simulink model "qrd_matrix_inversion"  (Simulink 8.7)
settings: Solver=VariableStepDiscrete  StartTime=0.0  StopTime=10  RelTol=1e-3
undefined symbols (not defined in the file or in its folder): dspba, Input_Fraction_Length, Input_Word_Length, value
libraries: DSPBAPrim x28, DSPBABase x6, qrd_matrix_library x1
Description:
  | DSP Builder Advanced Template for Template Design implementing Primitive Subsystems
settings Model: Creator=mjervis  LastModifiedBy=5g
settings DataIOCC: SignalLoggingSaveFormat=ModelDataLogs
settings OptimizationCC: ExpressionDepthLimit=2147483647
settings DebuggingCC: SolverPrmCheckMsg=warning  InheritedTsInSrcMsg=none  IntegerOverflowMsg=none  FcnCallInpInsideContextMsg=UseLocalSettings  AllowSymbolicDim=off  StateNameClashWarn=warning  IntegerSaturationMsg=none
settings GRTTargetCC: CombineOutputUpdateFcns=off  GRTInterface=on

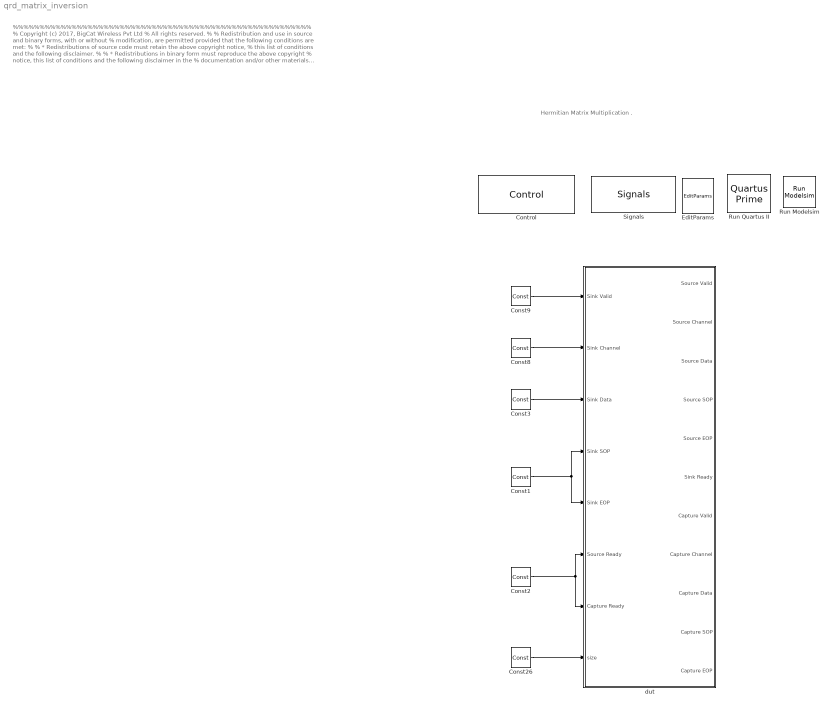
== system qrd_matrix_inversion ==
  note: %%%%%%%%%%%%%%%%%%%%%%%%%%%%%%%%%%%%%%%%%%%%%%%%%%%%%%%%
      |  % Copyright (c) 2017, BigCat Wireless Pvt Ltd
      |  % All rights reserved.
      |  %
      |  % Redistribution and use in source and binary forms, with or without
      |  % modification, are permitted provided that the following conditions are met:
      |  %
      |  %     * Redistributions of source code must retain the above copyright notice,
      |  %       this list of conditions and the following disclaimer.
      |  %
      |  %     * Redistributions in binary form must reproduce the above copyright
      |  %       notice, this list of conditions and the following disclaimer in the
      |  %       documentation and/or other materials provided with the distribution.
      |  %
      |  %     * Neither the name of the copyright holder nor the names of its contributors
      |  %       may be used to endorse or promote products derived from this software
      |  %       without specific prior written permission.
      |  %
      |  %
      |  %
      |  % THIS SOFTWARE IS PROVIDED BY THE COPYRIGHT HOLDERS AND CONTRIBUTORS "AS IS"
      |  % AND ANY EXPRESS OR IMPLIED WARRANTIES, INCLUDING, BUT NOT LIMITED TO, THE
      |  % IMPLIED WARRANTIES OF MERCHANTABILITY AND FITNESS FOR A PARTICULAR PURPOSE ARE
      |  % DISCLAIMED. IN NO EVENT SHALL THE COPYRIGHT HOLDER OR CONTRIBUTORS BE LIABLE
      |  % FOR ANY DIRECT, INDIRECT, INCIDENTAL, SPECIAL, EXEMPLARY, OR CONSEQUENTIAL
      |  % DAMAGES (INCLUDING, BUT NOT LIMITED TO, PROCUREMENT OF SUBSTITUTE GOODS OR
      |  % SERVICES; LOSS OF USE, DATA, OR PROFITS; OR BUSINESS INTERRUPTION) HOWEVER
      |  % CAUSED AND ON ANY THEORY OF LIABILITY, WHETHER IN CONTRACT, STRICT LIABILITY,
      |  % OR TORT (INCLUDING NEGLIGENCE OR OTHERWISE) ARISING IN ANY WAY OUT OF THE USE
      |  % OF THIS SOFTWARE, EVEN IF ADVISED OF THE POSSIBILITY OF SUCH DAMAGE.
      |  %
      |   %%%%%%%%%%%%%%%%%%%%%%%%%%%%%%%%%%%%%%%%%%%%%%%%%%%%%%%
  note: Hermitian Matrix Multiplication
      |                                                    .
  Const1 : DSPBAPrim/Const  primtype=const  nInputs=0  nOutputs=1  omode=boolean  otype=ufix(5)  scale=1  rndmethod=Unbiased  factor=1  satmethod=Symmetric  shift_vec=[0 1 2 -1]  value=0  inPortNames=['+'; '+';]  outPortNames=[' ']  dspbaimage=dspba_prim.jpg  text=fprintf('%s', num2str(value));  style=Optimised  visibilities=8 + 1024  floatPrecision=float32_m23  version=20120820
  Const2 : DSPBAPrim/Const  primtype=const  nInputs=0  nOutputs=1  omode=boolean  otype=ufix(5)  scale=1  rndmethod=Unbiased  factor=1  satmethod=Symmetric  shift_vec=[0 1 2 -1]  value=0  inPortNames=['+'; '+';]  outPortNames=[' ']  dspbaimage=dspba_prim.jpg  text=fprintf('%s', num2str(value));  style=Optimised  visibilities=8 + 1024  floatPrecision=float32_m23  version=20120820
  Const26 : DSPBAPrim/Const  primtype=const  nInputs=0  nOutputs=1  omode=Specify via dialog  otype=ufix(5)  scale=1  rndmethod=Unbiased  factor=1  satmethod=Symmetric  shift_vec=[0 1 2 -1]  value=16  inPortNames=['+'; '+';]  outPortNames=[' ']  dspbaimage=dspba_prim.jpg  text=fprintf('%s', num2str(value));  style=Optimised  visibilities=8 + 1024  floatPrecision=float32_m23  version=20120820
  Const3 : DSPBAPrim/Const  primtype=const  nInputs=0  nOutputs=1  omode=Specify via dialog  otype=uint(128)  scale=1  rndmethod=Unbiased  factor=1  satmethod=Symmetric  shift_vec=[0 1 2 -1]  value=0  inPortNames=['+'; '+';]  outPortNames=[' ']  dspbaimage=dspba_prim.jpg  text=fprintf('%s', num2str(value));  style=Optimised  visibilities=8 + 1024  floatPrecision=float32_m23  version=20120820
  Const8 : DSPBAPrim/Const  primtype=const  nInputs=0  nOutputs=1  omode=Specify via dialog  otype=uint(8)  scale=1  rndmethod=Unbiased  factor=1  satmethod=Symmetric  shift_vec=[0 1 2 -1]  value=0  inPortNames=['+'; '+';]  outPortNames=[' ']  dspbaimage=dspba_prim.jpg  text=fprintf('%s', num2str(value));  style=Optimised  visibilities=8 + 1024  floatPrecision=float32_m23  version=20120820
  Const9 : DSPBAPrim/Const  primtype=const  nInputs=0  nOutputs=1  omode=boolean  otype=uint(8)  scale=1  rndmethod=Unbiased  factor=1  satmethod=Symmetric  shift_vec=[0 1 2 -1]  value=0  inPortNames=['+'; '+';]  outPortNames=[' ']  dspbaimage=dspba_prim.jpg  text=fprintf('%s', num2str(value));  style=Optimised  visibilities=8 + 1024  floatPrecision=float32_m23  version=20120820
  Control : DSPBABase/Control  generate=on  language=VHDL  destination=./rtl  destination_gui=./rtl  make_full_path=off  path_is_relative=on  autotestbench=on  signaldepth=2  coveragetestbench=off  logs=off  spacewidth=2  spacenum=1  addrwidth=10  datawidth=16  dataendian=Big Endian  hierarchicalnames=off  ramThresholdBits=-1  distRamThresholdBits=500  mlabThresholdBits=-1  hardMultiplierThresholdLuts=-1  version=20090407  errorOnChanMismatch=1  errorOnGPIOMismatch=0  importModelsimResults=1  devOutputVar=vsimResults  verificationFunction=verify_qrd  cycleAccurate=off  reinterpretCastMult=off  paramFile=qrd_matrix_inversion_params.xml
  EditParams : DSPBABase/EditParams  version=20090407
  Run Modelsim : DSPBABase/Run Modelsim  version=20090407
  Run Quartus II : DSPBABase/Quartus Prime  version=20090407
  Signals : DSPBABase/Signals  clk=clk  freq=250  margin=0  rst=areset  rstactive=High  bus=bus  enbusclock=off  busfreq=250  bussync=off  version=20090407
  dut : Subsystem
  wires:
  Const2/1 -> dut/6(Source Ready), dut/7(Capture Ready)
  Const26/1 -> dut/8(size)
  Const1/1 -> dut/4(Sink SOP), dut/5(Sink EOP)
  Const3/1 -> dut/3(Sink Data)
  Const8/1 -> dut/2(Sink Channel)
  Const9/1 -> dut/1(Sink Valid)

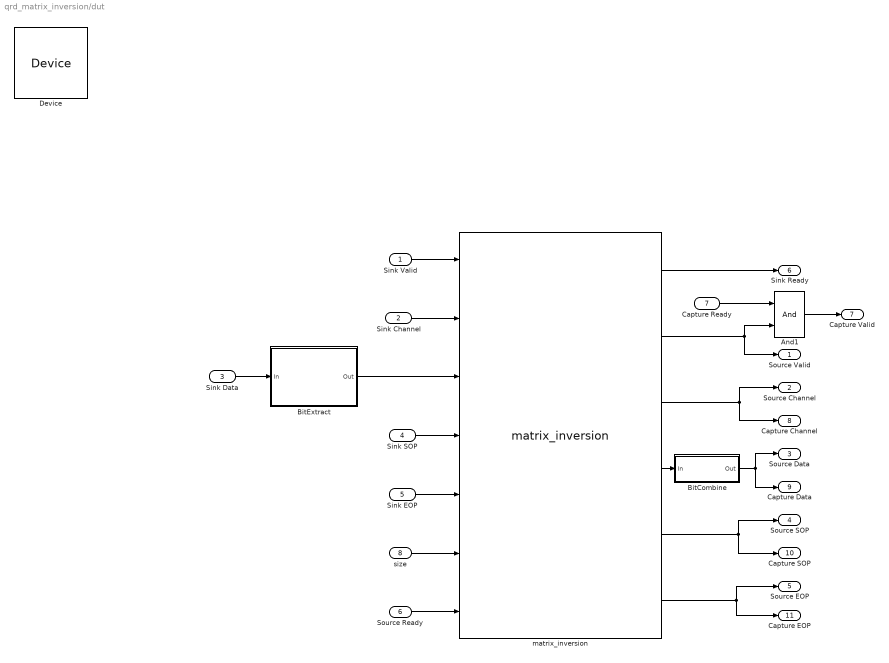
== system qrd_matrix_inversion/dut ==
  Sink Valid : Inport
  Sink Channel : Inport  Port=2
  Sink Data : Inport  Port=3
  Sink SOP : Inport  Port=4
  Sink EOP : Inport  Port=5
  Source Ready : Inport  Port=6
  Capture Ready : Inport  Port=7
  size : Inport  Port=8
  And1 : DSPBAPrim/And  primtype=and  nInputs=2  nOutputs=1  omode=Inherit via internal rule  otype=sfix(16)  scale=2^-15  rndmethod=Unbiased  factor=1  satmethod=Symmetric  shift_vec=[0 1 2 -1]  value=0  inPortNames=[' '; ' '; ' '; ' '; ' '; ' '; ' '; ' '; ' '; ' '; ' '; ' '; ' '; ' '; ' '; ' '; ]  outPortNames=[' ']  dspbaimage=dspba_prim.jpg  text=fprintf('&');  style=Optimised  visibilities=8+2  version=20090407
  BitCombine : Subsystem
  BitExtract : Subsystem
  Device : DSPBABase/Device  family=Arria 10  deviceMember=Arria 10  stratix4device=Stratix IV E  hardcopy4device=HardCopy IV E  stratix5device=Stratix V GX  device=10AS066N3F40E2SGE2  speed=2  stratixSpeed=-5  stratix2Speed=-3  stratix3Speed=-2  stratix4gxSpeed=-2  stratix4gtSpeed=-1  cyclone2Speed=-6  cyclone3Speed=-7  arria2Speed=-4  cyclone4eSpeed=-8  stratix5Speed=-3  arria5Speed=-4  arriaSpeed=-6  cyclone3lsSpeed=-7  cyclone5Speed=-6  arria2gzSpeed=-3  nightFurySpeed=-2  ecp2Speed=-7  hardcopycompat=off  version=20140217  max10flashmode=off  max10nomeminit=off
  matrix_inversion : qrd_matrix_library/matrix_inversion  size=16  QRD_vectorization=2  Back_Substitution_instances=4
      link override Back_Substitution: SourceBlock=qrd_matrix_library/Back_Substitution
      link override Back_Substitution/Channel Latch: SourceBlock=qrd_matrix_library/Latch
      link override Back_Substitution/Channel Latch/ChannelOut: latency=0
      link override Back_Substitution/Control Logic/Rising Edge Detect: SourceBlock=qrd_matrix_library/matrix_multiplication/Rising Edge Detect
      link override Back_Substitution/Control Logic/Rising Edge Detect1: SourceBlock=qrd_matrix_library/matrix_multiplication/Rising Edge Detect
      link override Back_Substitution/Data Mux/ChannelOut: latency=2
      link override Back_Substitution/Dot Product/Dot Product ChannelOut: latency=16
      link override Back_Substitution/Dot Product/Mult ChannelOut: latency=9
      link override Back_Substitution/Latch: SourceBlock=qrd_matrix_library/Latch
      link override Back_Substitution/Latch/ChannelOut: latency=1
      link override Back_Substitution/Mult/ChannelOut: latency=7
      link override Back_Substitution/Rising Edge Detect: SourceBlock=qrd_matrix_library/matrix_multiplication/Rising Edge Detect
      link override Back_Substitution/Sub/ChannelOut: latency=3
      link override Channel Latch: SourceBlock=qrd_matrix_library/Latch
      link override Channel Latch/ChannelOut: latency=1
      link override Conjugate/ChannelOut: latency=2
      link override QR_decomposition: SourceBlock=qrd_matrix_library/QR_decomposition
      link override QR_decomposition/A_j/ChannelOut: latency=4
      link override QR_decomposition/Channel Latch: SourceBlock=qrd_matrix_library/Latch
      link override QR_decomposition/Channel Latch/ChannelOut: latency=1
      link override QR_decomposition/Control Logic/A_j_Address_Gen/ChannelOut: latency=3
      link override QR_decomposition/Control Logic/A_k_Address_Gen/ChannelOut: latency=3
      link override QR_decomposition/Control Logic/Rising Edge Detect: SourceBlock=qrd_matrix_library/hermitian_matrix_multiplication/Rising Edge Detect
      link override QR_decomposition/Control Logic/Rising Edge Detect1: SourceBlock=qrd_matrix_library/hermitian_matrix_multiplication/Rising Edge Detect
      link override QR_decomposition/Control Logic/Rising Edge Detect2: SourceBlock=qrd_matrix_library/hermitian_matrix_multiplication/Rising Edge Detect
      link override QR_decomposition/Control Logic/Rising Edge Detect3: SourceBlock=qrd_matrix_library/hermitian_matrix_multiplication/Rising Edge Detect
      link override QR_decomposition/Control Logic/Rising Edge Detect4: SourceBlock=qrd_matrix_library/hermitian_matrix_multiplication/Rising Edge Detect
      link override QR_decomposition/Control Logic/rn_k_j_Address_Gen/ChannelOut: latency=3
      link override QR_decomposition/Data Mux/ChannelOut: latency=4
      link override QR_decomposition/Dot Product/Dot Product ChannelOut: latency=20
      link override QR_decomposition/Dot Product/Mult ChannelOut: latency=9
      link override QR_decomposition/Inv SQRT/inv_r2_k_k ChannelOut: latency=15
      link override QR_decomposition/Inv SQRT/inv_r_k_k ChannelOut: latency=11
      link override QR_decomposition/Inv_Rk Output Memory Controller/Rising Edge Detect: SourceBlock=qrd_matrix_library/matrix_multiplication/Rising Edge Detect
      link override QR_decomposition/Latch: SourceBlock=qrd_matrix_library/Latch
      link override QR_decomposition/Latch/ChannelOut: latency=1
      link override QR_decomposition/Q Output Memory Controller/Rising Edge Detect: SourceBlock=qrd_matrix_library/matrix_multiplication/Rising Edge Detect
      link override QR_decomposition/Rising Edge Detect3: SourceBlock=qrd_matrix_library/hermitian_matrix_multiplication/Rising Edge Detect
      link override QR_decomposition/Rn Output Memory Controller/Rising Edge Detect: SourceBlock=qrd_matrix_library/matrix_multiplication/Rising Edge Detect
      link override QR_decomposition/rk/ChannelOut: latency=3
      link override QR_decomposition/rn_k_j_over_r2_k_k/ChannelOut: latency=3
      link override Rising Edge Detect3: SourceBlock=qrd_matrix_library/hermitian_matrix_multiplication/Rising Edge Detect
      link override Z_Address_Gen/Add: otype=uint(nextpow2(size*size/Back_Substitution_instances))
      link override Z_Address_Gen/ChannelOut: latency=3
      link override vectorizer/ChannelOut: latency=1
      link override vectorizer/TappedDelay: SourceBlock=qrd_matrix_library/TappedDelay
  Source Valid : Outport
  Source Channel : Outport  Port=2
  Source Data : Outport  Port=3
  Source SOP : Outport  Port=4
  Source EOP : Outport  Port=5
  Sink Ready : Outport  Port=6
  Capture Valid : Outport  Port=7
  Capture Channel : Outport  Port=8
  Capture Data : Outport  Port=9
  Capture SOP : Outport  Port=10
  Capture EOP : Outport  Port=11
  wires:
  Capture Ready/1 -> And1/1
  And1/1 -> Capture Valid/1
  matrix_inversion/1 -> Sink Ready/1
  size/1 -> matrix_inversion/6
  matrix_inversion/6 -> Source EOP/1, Capture EOP/1
  matrix_inversion/3 -> Source Channel/1, Capture Channel/1
  matrix_inversion/2 -> Source Valid/1, And1/2
  Sink Valid/1 -> matrix_inversion/1
  Sink Channel/1 -> matrix_inversion/2
  Sink SOP/1 -> matrix_inversion/4
  Sink EOP/1 -> matrix_inversion/5
  Sink Data/1 -> BitExtract/1(In)
  BitExtract/1(Out) -> matrix_inversion/3
  BitCombine/1(Out) -> Source Data/1, Capture Data/1
  matrix_inversion/4 -> BitCombine/1(In)
  Source Ready/1 -> matrix_inversion/7
  matrix_inversion/5 -> Source SOP/1, Capture SOP/1

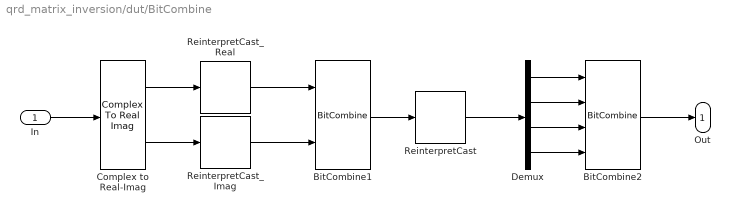
== system qrd_matrix_inversion/dut/BitCombine ==
  In : Inport
  BitCombine1 : DSPBAPrim/BitCombine  primtype=bitcombine  nInputs=2  nOutputs=1  omode=Specify via dialog  otype=uint(64)  scale=1  rndmethod=Unbiased  factor=1  satmethod=Symmetric  shift_vec=[0 1 2 -1]  value=0  inPortNames=['l'; 'h';]  outPortNames=[' ']  dspbaimage=dspba_prim.jpg  text=fprintf('[h,l]');  style=Optimised  visibilities=8+2  version=20090407
  BitCombine2 : DSPBAPrim/BitCombine  primtype=bitcombine  nInputs=4  nOutputs=1  omode=Specify via dialog  otype=uint(256)  scale=1  rndmethod=Unbiased  factor=1  satmethod=Symmetric  shift_vec=[0 1 2 -1]  value=0  inPortNames=['l'; 'h';]  outPortNames=[' ']  dspbaimage=dspba_prim.jpg  text=fprintf('[h,l]');  style=Optimised  visibilities=8+2  version=20090407
  Complex to Real-Imag : ComplexToRealImag
  Demux : Demux
  ReinterpretCast : DSPBAPrim/ReinterpretCast  primtype=reinterpret  nInputs=1  nOutputs=1  omode=Specify via dialog  otype=uint(64)  scale=1  rndmethod=Unbiased  factor=1  satmethod=Symmetric  shift_vec=[0 1 2 -1]  value=0  inPortNames=[' '; ' ';]  outPortNames=[' ']  dspbaimage=dspba_prim.jpg  text=fprintf('Reinterp\nCast', value);  style=Optimised  visibilities=8  floatPrecision=float32_m23  version=20120601
  ReinterpretCast_Imag : DSPBAPrim/ReinterpretCast  primtype=reinterpret  nInputs=1  nOutputs=1  omode=Specify via dialog  otype=uint(32)  scale=1  rndmethod=Unbiased  factor=1  satmethod=Symmetric  shift_vec=[0 1 2 -1]  value=0  inPortNames=[' '; ' ';]  outPortNames=[' ']  dspbaimage=dspba_prim.jpg  text=fprintf('Reinterp\nCast', value);  style=Optimised  visibilities=8  floatPrecision=float32_m23  version=20120601
  ReinterpretCast_Real : DSPBAPrim/ReinterpretCast  primtype=reinterpret  nInputs=1  nOutputs=1  omode=Specify via dialog  otype=uint(32)  scale=1  rndmethod=Unbiased  factor=1  satmethod=Symmetric  shift_vec=[0 1 2 -1]  value=0  inPortNames=[' '; ' ';]  outPortNames=[' ']  dspbaimage=dspba_prim.jpg  text=fprintf('Reinterp\nCast', value);  style=Optimised  visibilities=8  floatPrecision=float32_m23  version=20120601
  Out : Outport
  wires:
  Complex to Real-Imag/1 -> ReinterpretCast_Real/1
  Complex to Real-Imag/2 -> ReinterpretCast_Imag/1
  BitCombine1/1 -> ReinterpretCast/1
  ReinterpretCast_Real/1 -> BitCombine1/1
  ReinterpretCast_Imag/1 -> BitCombine1/2
  In/1 -> Complex to Real-Imag/1
  ReinterpretCast/1 -> Demux/1
  Demux/4 -> BitCombine2/4
  Demux/3 -> BitCombine2/3
  Demux/2 -> BitCombine2/2
  Demux/1 -> BitCombine2/1
  BitCombine2/1 -> Out/1

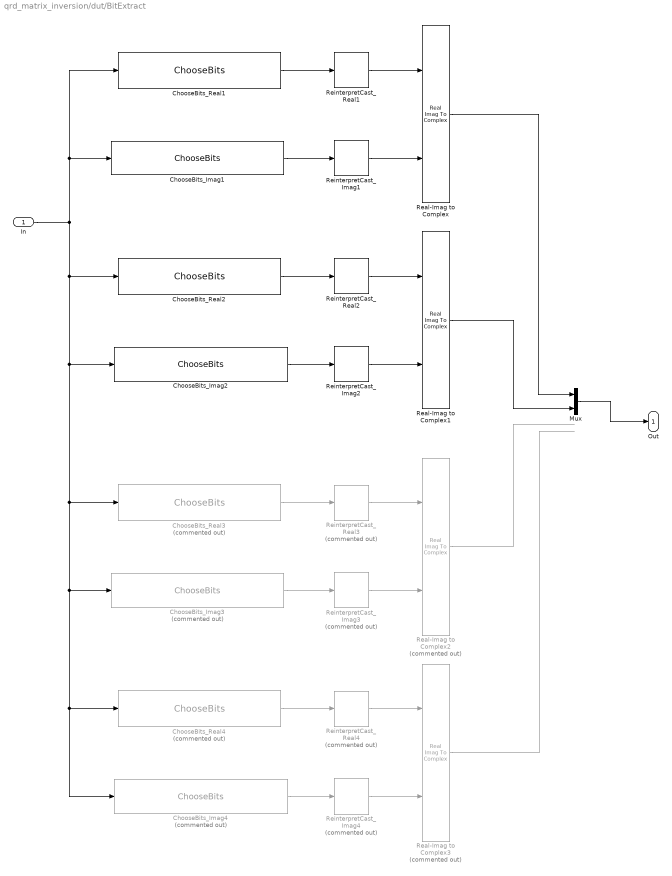
== system qrd_matrix_inversion/dut/BitExtract ==
  In : Inport
  ChooseBits_Imag1 : DSPBAPrim/ChooseBits  primtype=choosebits  nInputs=1  nOutputs=1  omode=Inherit via internal rule  otype=fixdt(0,1,1)  scale=1  rndmethod=Unbiased  factor=1  satmethod=Symmetric  shift_vec=[0 1 2 -1]  value=[32:63]  inPortNames=[' '; ' ';]  outPortNames=[' ']  dspbaimage=dspba_prim.jpg  text=fprintf('%s',dspba.perm2str(value));  style=Optimised  visibilities=1024  version=20090407
  ChooseBits_Imag2 : DSPBAPrim/ChooseBits  primtype=choosebits  nInputs=1  nOutputs=1  omode=Inherit via internal rule  otype=fixdt(0,1,1)  scale=1  rndmethod=Unbiased  factor=1  satmethod=Symmetric  shift_vec=[0 1 2 -1]  value=[96:127]  inPortNames=[' '; ' ';]  outPortNames=[' ']  dspbaimage=dspba_prim.jpg  text=fprintf('%s',dspba.perm2str(value));  style=Optimised  visibilities=1024  version=20090407
  ChooseBits_Imag3 : DSPBAPrim/ChooseBits  Commented=on  primtype=choosebits  nInputs=1  nOutputs=1  omode=Inherit via internal rule  otype=fixdt(0,1,1)  scale=1  rndmethod=Unbiased  factor=1  satmethod=Symmetric  shift_vec=[0 1 2 -1]  value=[160:191]  inPortNames=[' '; ' ';]  outPortNames=[' ']  dspbaimage=dspba_prim.jpg  text=fprintf('%s',dspba.perm2str(value));  style=Optimised  visibilities=1024  version=20090407
  ChooseBits_Imag4 : DSPBAPrim/ChooseBits  Commented=on  primtype=choosebits  nInputs=1  nOutputs=1  omode=Inherit via internal rule  otype=fixdt(0,1,1)  scale=1  rndmethod=Unbiased  factor=1  satmethod=Symmetric  shift_vec=[0 1 2 -1]  value=[224:255]  inPortNames=[' '; ' ';]  outPortNames=[' ']  dspbaimage=dspba_prim.jpg  text=fprintf('%s',dspba.perm2str(value));  style=Optimised  visibilities=1024  version=20090407
  ChooseBits_Real1 : DSPBAPrim/ChooseBits  primtype=choosebits  nInputs=1  nOutputs=1  omode=Inherit via internal rule  otype=fixdt(0,1,1)  scale=1  rndmethod=Unbiased  factor=1  satmethod=Symmetric  shift_vec=[0 1 2 -1]  value=[0:31]  inPortNames=[' '; ' ';]  outPortNames=[' ']  dspbaimage=dspba_prim.jpg  text=fprintf('%s',dspba.perm2str(value));  style=Optimised  visibilities=1024  version=20090407
  ChooseBits_Real2 : DSPBAPrim/ChooseBits  primtype=choosebits  nInputs=1  nOutputs=1  omode=Inherit via internal rule  otype=fixdt(0,1,1)  scale=1  rndmethod=Unbiased  factor=1  satmethod=Symmetric  shift_vec=[0 1 2 -1]  value=[64:95]  inPortNames=[' '; ' ';]  outPortNames=[' ']  dspbaimage=dspba_prim.jpg  text=fprintf('%s',dspba.perm2str(value));  style=Optimised  visibilities=1024  version=20090407
  ChooseBits_Real3 : DSPBAPrim/ChooseBits  Commented=on  primtype=choosebits  nInputs=1  nOutputs=1  omode=Inherit via internal rule  otype=fixdt(0,1,1)  scale=1  rndmethod=Unbiased  factor=1  satmethod=Symmetric  shift_vec=[0 1 2 -1]  value=[128:159]  inPortNames=[' '; ' ';]  outPortNames=[' ']  dspbaimage=dspba_prim.jpg  text=fprintf('%s',dspba.perm2str(value));  style=Optimised  visibilities=1024  version=20090407
  ChooseBits_Real4 : DSPBAPrim/ChooseBits  Commented=on  primtype=choosebits  nInputs=1  nOutputs=1  omode=Inherit via internal rule  otype=fixdt(0,1,1)  scale=1  rndmethod=Unbiased  factor=1  satmethod=Symmetric  shift_vec=[0 1 2 -1]  value=[192:223]  inPortNames=[' '; ' ';]  outPortNames=[' ']  dspbaimage=dspba_prim.jpg  text=fprintf('%s',dspba.perm2str(value));  style=Optimised  visibilities=1024  version=20090407
  Mux : Mux  Inputs=2
  Real-Imag to Complex : RealImagToComplex
  Real-Imag to Complex1 : RealImagToComplex
  Real-Imag to Complex2 : RealImagToComplex  Commented=on
  Real-Imag to Complex3 : RealImagToComplex  Commented=on
  ReinterpretCast_Imag1 : DSPBAPrim/ReinterpretCast  primtype=reinterpret  nInputs=1  nOutputs=1  omode=single  otype=sfix(Input_Word_Length)  scale=2^-(Input_Fraction_Length)  rndmethod=Unbiased  factor=1  satmethod=Symmetric  shift_vec=[0 1 2 -1]  value=0  inPortNames=[' '; ' ';]  outPortNames=[' ']  dspbaimage=dspba_prim.jpg  text=fprintf('Reinterp\nCast', value);  style=Optimised  visibilities=8  floatPrecision=float32_m23  version=20120601
  ReinterpretCast_Imag2 : DSPBAPrim/ReinterpretCast  primtype=reinterpret  nInputs=1  nOutputs=1  omode=single  otype=sfix(Input_Word_Length)  scale=2^-(Input_Fraction_Length)  rndmethod=Unbiased  factor=1  satmethod=Symmetric  shift_vec=[0 1 2 -1]  value=0  inPortNames=[' '; ' ';]  outPortNames=[' ']  dspbaimage=dspba_prim.jpg  text=fprintf('Reinterp\nCast', value);  style=Optimised  visibilities=8  floatPrecision=float32_m23  version=20120601
  ReinterpretCast_Imag3 : DSPBAPrim/ReinterpretCast  Commented=on  primtype=reinterpret  nInputs=1  nOutputs=1  omode=single  otype=sfix(Input_Word_Length)  scale=2^-(Input_Fraction_Length)  rndmethod=Unbiased  factor=1  satmethod=Symmetric  shift_vec=[0 1 2 -1]  value=0  inPortNames=[' '; ' ';]  outPortNames=[' ']  dspbaimage=dspba_prim.jpg  text=fprintf('Reinterp\nCast', value);  style=Optimised  visibilities=8  floatPrecision=float32_m23  version=20120601
  ReinterpretCast_Imag4 : DSPBAPrim/ReinterpretCast  Commented=on  primtype=reinterpret  nInputs=1  nOutputs=1  omode=single  otype=sfix(Input_Word_Length)  scale=2^-(Input_Fraction_Length)  rndmethod=Unbiased  factor=1  satmethod=Symmetric  shift_vec=[0 1 2 -1]  value=0  inPortNames=[' '; ' ';]  outPortNames=[' ']  dspbaimage=dspba_prim.jpg  text=fprintf('Reinterp\nCast', value);  style=Optimised  visibilities=8  floatPrecision=float32_m23  version=20120601
  ReinterpretCast_Real1 : DSPBAPrim/ReinterpretCast  primtype=reinterpret  nInputs=1  nOutputs=1  omode=single  otype=sfix(Input_Word_Length)  scale=2^-(Input_Fraction_Length)  rndmethod=Unbiased  factor=1  satmethod=Symmetric  shift_vec=[0 1 2 -1]  value=0  inPortNames=[' '; ' ';]  outPortNames=[' ']  dspbaimage=dspba_prim.jpg  text=fprintf('Reinterp\nCast', value);  style=Optimised  visibilities=8  floatPrecision=float32_m23  version=20120601
  ReinterpretCast_Real2 : DSPBAPrim/ReinterpretCast  primtype=reinterpret  nInputs=1  nOutputs=1  omode=single  otype=sfix(Input_Word_Length)  scale=2^-(Input_Fraction_Length)  rndmethod=Unbiased  factor=1  satmethod=Symmetric  shift_vec=[0 1 2 -1]  value=0  inPortNames=[' '; ' ';]  outPortNames=[' ']  dspbaimage=dspba_prim.jpg  text=fprintf('Reinterp\nCast', value);  style=Optimised  visibilities=8  floatPrecision=float32_m23  version=20120601
  ReinterpretCast_Real3 : DSPBAPrim/ReinterpretCast  Commented=on  primtype=reinterpret  nInputs=1  nOutputs=1  omode=single  otype=sfix(Input_Word_Length)  scale=2^-(Input_Fraction_Length)  rndmethod=Unbiased  factor=1  satmethod=Symmetric  shift_vec=[0 1 2 -1]  value=0  inPortNames=[' '; ' ';]  outPortNames=[' ']  dspbaimage=dspba_prim.jpg  text=fprintf('Reinterp\nCast', value);  style=Optimised  visibilities=8  floatPrecision=float32_m23  version=20120601
  ReinterpretCast_Real4 : DSPBAPrim/ReinterpretCast  Commented=on  primtype=reinterpret  nInputs=1  nOutputs=1  omode=single  otype=sfix(Input_Word_Length)  scale=2^-(Input_Fraction_Length)  rndmethod=Unbiased  factor=1  satmethod=Symmetric  shift_vec=[0 1 2 -1]  value=0  inPortNames=[' '; ' ';]  outPortNames=[' ']  dspbaimage=dspba_prim.jpg  text=fprintf('Reinterp\nCast', value);  style=Optimised  visibilities=8  floatPrecision=float32_m23  version=20120601
  Out : Outport
  wires:
  ReinterpretCast_Real1/1 -> Real-Imag to Complex/1
  ReinterpretCast_Real2/1 -> Real-Imag to Complex1/1
  ChooseBits_Real2/1 -> ReinterpretCast_Real2/1
  ChooseBits_Real1/1 -> ReinterpretCast_Real1/1
  ReinterpretCast_Imag2/1 -> Real-Imag to Complex1/2
  ReinterpretCast_Imag1/1 -> Real-Imag to Complex/2
  ChooseBits_Imag1/1 -> ReinterpretCast_Imag1/1
  ChooseBits_Imag2/1 -> ReinterpretCast_Imag2/1
  Mux/1 -> Out/1
  Real-Imag to Complex1/1 -> Mux/2
  Real-Imag to Complex/1 -> Mux/1
  In/1 -> ChooseBits_Imag1/1, ChooseBits_Real1/1, ChooseBits_Real2/1, ChooseBits_Real4/1, ChooseBits_Imag4/1, ChooseBits_Imag3/1, ChooseBits_Real3/1, ChooseBits_Imag2/1
  ReinterpretCast_Real3/1 -> Real-Imag to Complex2/1
  ReinterpretCast_Real4/1 -> Real-Imag to Complex3/1
  ChooseBits_Real4/1 -> ReinterpretCast_Real4/1
  ChooseBits_Real3/1 -> ReinterpretCast_Real3/1
  ReinterpretCast_Imag4/1 -> Real-Imag to Complex3/2
  ReinterpretCast_Imag3/1 -> Real-Imag to Complex2/2
  ChooseBits_Imag3/1 -> ReinterpretCast_Imag3/1
  ChooseBits_Imag4/1 -> ReinterpretCast_Imag4/1
  Real-Imag to Complex2/1 -> ?
  Real-Imag to Complex3/1 -> ?
